simulink model "nelinerani_i_linearni_model_neupravljanog_objekta"  (R2018a)
settings: Solver=ode4  StartTime=0.0  StopTime=700  FixedStep=0.01  RelTol=1e-3  EnableMultiTasking=on
values from neighbouring files (symbols this model uses):
  Ar1 = 0.04    [skript_prvi_deo.m]
  Ar2 = 0.04    [skript_prvi_deo.m]
  Cd1 = 0.65    [skript_prvi_deo.m]
  Cd2 = 0.65    [skript_prvi_deo.m]
  Cdh = 0.65    [skript_prvi_deo.m]
  Cdt = 0.65    [skript_prvi_deo.m]
  df1_H1 = double(subs(df1_H1, [Uvt Uvh Uv2 Pt H1 H2 theta_m], [Uvt_N Uvh_N Uv2_N Pt_N H1_N H2_N theta_m_N]))    [skript_prvi_deo.m]
  df1_Pt = double(subs(df1_Pt, [Uvt Uvh Uv2 Pt H1 H2 theta_m], [Uvt_N Uvh_N Uv2_N Pt_N H1_N H2_N theta_m_N]))    [skript_prvi_deo.m]
  df1_Uvh = double(subs(df1_Uvh, [Uvt Uvh Uv2 Pt H1 H2 theta_m], [Uvt_N Uvh_N Uv2_N Pt_N H1_N H2_N theta_m_N]))    [skript_prvi_deo.m]
  df1_Uvt = double(subs(df1_Uvt, [Uvt Uvh Uv2 Pt H1 H2 theta_m], [Uvt_N Uvh_N Uv2_N Pt_N H1_N H2_N theta_m_N]))    [skript_prvi_deo.m]
  df2_H1 = double(subs(df2_H1, [Uvt Uvh Uv2 Pt H1 H2 theta_m], [Uvt_N Uvh_N Uv2_N Pt_N H1_N H2_N theta_m_N]))    [skript_prvi_deo.m]
  df2_H2 = double(subs(df2_H2, [Uvt Uvh Uv2 Pt H1 H2 theta_m], [Uvt_N Uvh_N Uv2_N Pt_N H1_N H2_N theta_m_N]))    [skript_prvi_deo.m]
  df2_Uv2 = double(subs(df2_Uv2, [Uvt Uvh Uv2 Pt H1 H2 theta_m], [Uvt_N Uvh_N Uv2_N Pt_N H1_N H2_N theta_m_N]))    [skript_prvi_deo.m]
  df3_H1 = double(subs(df3_H1, [Uvt Uvh Uv2 Pt H1 H2 theta_m], [Uvt_N Uvh_N Uv2_N Pt_N H1_N H2_N theta_m_N]))    [skript_prvi_deo.m]
  df3_Pt = double(subs(df3_Pt, [Uvt Uvh Uv2 Pt H1 H2 theta_m], [Uvt_N Uvh_N Uv2_N Pt_N H1_N H2_N theta_m_N]))    [skript_prvi_deo.m]
  df3_theta_m = double(subs(df3_theta_m, [Uvt Uvh Uv2 Pt H1 H2 theta_m], [Uvt_N Uvh_N Uv2_N Pt_N H1_N H2_N theta_m_N]))    [skript_prvi_deo.m]
  df3_Uvh = double(subs(df3_Uvh, [Uvt Uvh Uv2 Pt H1 H2 theta_m], [Uvt_N Uvh_N Uv2_N Pt_N H1_N H2_N theta_m_N]))    [skript_prvi_deo.m]
  df3_Uvt = double(subs(df3_Uvt, [Uvt Uvh Uv2 Pt H1 H2 theta_m], [Uvt_N Uvh_N Uv2_N Pt_N H1_N H2_N theta_m_N]))    [skript_prvi_deo.m]
  g = 9.81    [skript_prvi_deo.m]
  H1_max = 1.5    [skript_prvi_deo.m]
  H1_min = 0    [skript_prvi_deo.m]
  H1_N = 0.7    [skript_prvi_deo.m]
  H2_max = 1.5    [skript_prvi_deo.m]
  H2_min = 0    [skript_prvi_deo.m]
  H2_N = 0.8    [skript_prvi_deo.m]
  Kv1 = 1.5/1000    (= 0.0015)    [skript_prvi_deo.m]
  Kv2 = 1.5/1000    (= 0.0015)    [skript_prvi_deo.m]
  Kvh = 1/1000    (= 0.001)    [skript_prvi_deo.m]
  Kvt = 1/1000    (= 0.001)    [skript_prvi_deo.m]
  Ph = 3.25*10^5    (= 325000)    [skript_prvi_deo.m]
  Pt_N = 3.25*10^5    (= 325000)    [skript_prvi_deo.m]
  ro = 1000    [skript_prvi_deo.m]
  theta_h = 10 + 273    (= 283)    [skript_prvi_deo.m]
  theta_m_N = 30 + 273    (= 303)    [skript_prvi_deo.m]
  theta_t = 70 + 273    (= 343)    [skript_prvi_deo.m]
  Uv1 = 3    [skript_prvi_deo.m]
  Uv2_max = 10    [skript_prvi_deo.m]
  Uv2_min = 0    [skript_prvi_deo.m]
  Uv2_N = double(solve(e3 == 0, U2_N))    [skript_prvi_deo.m]
  Uvh_max = 10    [skript_prvi_deo.m]
  Uvh_min = 0    [skript_prvi_deo.m]
  Uvh_N = double(solve(f1n == 0, Uh_N))    [skript_prvi_deo.m]
  Uvt_max = 10    [skript_prvi_deo.m]
  Uvt_min = 0    [skript_prvi_deo.m]
  Uvt_N = double(solve(sol1 == sol2, Uvt_N))    [skript_prvi_deo.m]
  w1 = 0.1    [skript_prvi_deo.m]
  w2 = 0.1    [skript_prvi_deo.m]
  wh = 0.03    [skript_prvi_deo.m]
  wt = 0.03    [skript_prvi_deo.m]
settings Model: Creator=Nikola  LastModifiedBy=lakim
settings DataIOCC: LimitDataPoints=on  SaveFormat=Array
settings OptimizationCC: LifeSpan=inf
settings DebuggingCC: SFUnexpectedBacktrackingDiag=warning  SFNoUnconditionalDefaultTransitionDiag=warning  SFExecutionAtInitializationDiag=none
settings HardwareCC: ProdBitPerPointer=32  ProdBitPerSizeT=32  ProdBitPerPtrDiffT=32  ProdLargestAtomicFloat=None  ProdIntDivRoundTo=Undefined  ProdEndianess=Unspecified  ProdWordSize=32  ProdHWDeviceType=32-bit Generic
settings ModelReferenceCC: PropagateSignalLabelsOutOfModel=off
settings CodeAppCC: StateflowObjectComments=on
settings GRTTargetCC: TargetLangStandard=C89/C90 (ANSI)  GeneratePreprocessorConditionals=Disable all
settings ConfigComp: CovMetricSettings=dw  CovHtmlReporting=on  CovSaveCumulativeToWorkspaceVar=on  CovSaveSingleToWorkspaceVar=on  CovExternalEMLEnable=off

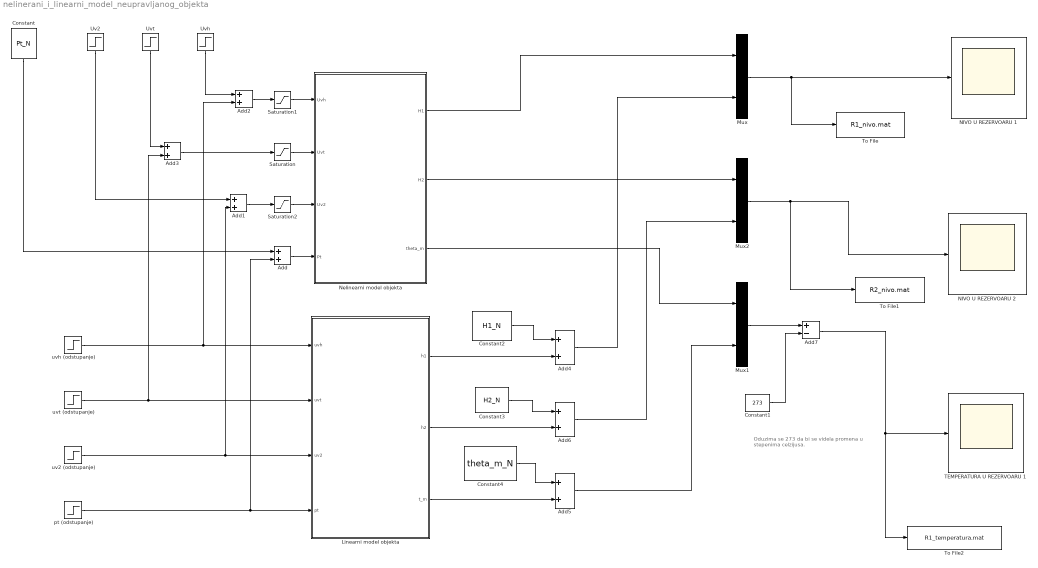
== system nelinerani_i_linearni_model_neupravljanog_objekta ==
  note: Oduzima se 273 da
      | bi se videla promena
      | u stepenima celzijusa.
  Add{,1..6} (7 alike) : Sum
  Add7 : Sum  Inputs=+-
  Constant : Constant  Value=Pt_N
  Constant1 : Constant  Value=273
  Constant2 : Constant  Value=H1_N
  Constant3 : Constant  Value=H2_N
  Constant4 : Constant  Value=theta_m_N
  Linearni model objekta : Subsystem
  Mux : Mux  Inputs=2
  Mux1 : Mux  Inputs=2
  Mux2 : Mux  Inputs=2
  NIVO U REZERVOARU 1 : Scope
  NIVO U REZERVOARU 2 : Scope
  Nelinearni model objekta : Subsystem
  Saturation : Saturate  UpperLimit=Uvt_max  LowerLimit=Uvt_min
  Saturation1 : Saturate  UpperLimit=Uvh_max  LowerLimit=Uvh_min
  Saturation2 : Saturate  UpperLimit=Uv2_max  LowerLimit=Uv2_min
  TEMPERATURA U REZERVOARU 1 : Scope
  To File : ToFile  Filename=R1_nivo.mat  MatrixName=H1
  To File1 : ToFile  Filename=R2_nivo.mat  MatrixName=H2
  To File2 : ToFile  Filename=R1_temperatura.mat  MatrixName=theta
  Uv2 : Step  Time=0  After=Uv2_N  SampleTime=0
  Uvh : Step  Time=0  After=Uvh_N  SampleTime=0
  Uvt : Step  Time=0  After=Uvt_N  SampleTime=0
  pt (odstupanje) : Step  Time=0  After=10^3  SampleTime=0
  uv2 (odstupanje) : Step  Time=0  After=0  SampleTime=0
  uvh (odstupanje) : Step  Time=150  After=0.1  SampleTime=0
  uvt (odstupanje) : Step  Time=0  After=0  SampleTime=0
  wires:
  Constant/1 -> Add/1
  Add3/1 -> Saturation/1
  Uvt/1 -> Add3/1
  Uvh/1 -> Add2/1
  Uv2/1 -> Add1/1
  Nelinearni model objekta/1(H1) -> Mux/1
  Mux/1 -> To File/1, NIVO U REZERVOARU 1/1
  Nelinearni model objekta/2(H2) -> Mux2/1
  Mux2/1 -> To File1/1, NIVO U REZERVOARU 2/1
  Nelinearni model objekta/3(theta_m) -> Mux1/1
  Add2/1 -> Saturation1/1
  Saturation/1 -> Nelinearni model objekta/2(Uvt)
  Add1/1 -> Saturation2/1
  uvh (odstupanje)/1 -> Add2/2, Linearni model objekta/1(uvh)
  uvt (odstupanje)/1 -> Add3/2, Linearni model objekta/2(uvt)
  uv2 (odstupanje)/1 -> Linearni model objekta/3(uv2), Add1/2
  pt (odstupanje)/1 -> Linearni model objekta/4(pt), Add/2
  Linearni model objekta/1(h1) -> Add4/2
  Linearni model objekta/2(h2) -> Add6/2
  Linearni model objekta/3(t_m) -> Add5/2
  Constant4/1 -> Add5/1
  Constant3/1 -> Add6/1
  Constant2/1 -> Add4/1
  Add4/1 -> Mux/2
  Add6/1 -> Mux2/2
  Add5/1 -> Mux1/2
  Add/1 -> Nelinearni model objekta/4(Pt)
  Saturation1/1 -> Nelinearni model objekta/1(Uvh)
  Saturation2/1 -> Nelinearni model objekta/3(Uv2)
  Mux1/1 -> Add7/1
  Add7/1 -> To File2/1, TEMPERATURA U REZERVOARU 1/1
  Constant1/1 -> Add7/2

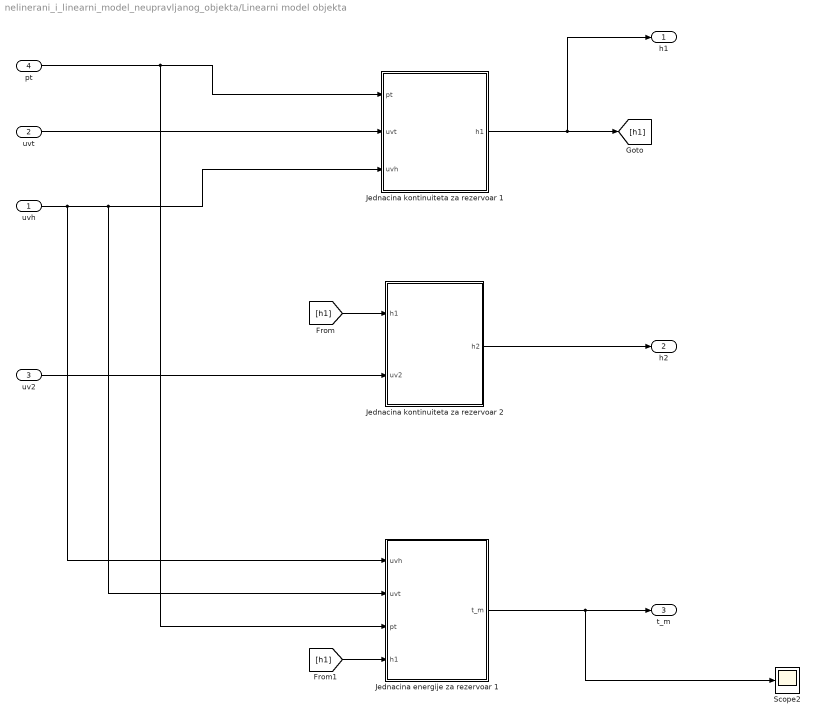
== system nelinerani_i_linearni_model_neupravljanog_objekta/Linearni model objekta ==
  uvh : Inport
  uvt : Inport  Port=2
  uv2 : Inport  Port=3
  pt : Inport  Port=4
  Jednacina energije za rezervoar 1 : Subsystem
  Jednacina kontinuiteta za rezervoar 1 : Subsystem
  Jednacina kontinuiteta za rezervoar 2 : Subsystem
  Scope2 : Scope
  h1 : Outport
  h2 : Outport  Port=2
  t_m : Outport  Port=3
  wires:
  Jednacina kontinuiteta za rezervoar 1/1(h1) -> h1/1, [h1]
  [h1] -> Jednacina kontinuiteta za rezervoar 2/1(h1)
  Jednacina kontinuiteta za rezervoar 2/1(h2) -> h2/1
  Jednacina energije za rezervoar 1/1(t_m) -> Scope2/1, t_m/1
  pt/1 -> Jednacina energije za rezervoar 1/3(pt), Jednacina kontinuiteta za rezervoar 1/1(pt)
  uvt/1 -> Jednacina kontinuiteta za rezervoar 1/2(uvt)
  uvh/1 -> Jednacina energije za rezervoar 1/1(uvh), Jednacina energije za rezervoar 1/2(uvt), Jednacina kontinuiteta za rezervoar 1/3(uvh)
  uv2/1 -> Jednacina kontinuiteta za rezervoar 2/2(uv2)
  [h1] -> Jednacina energije za rezervoar 1/4(h1)

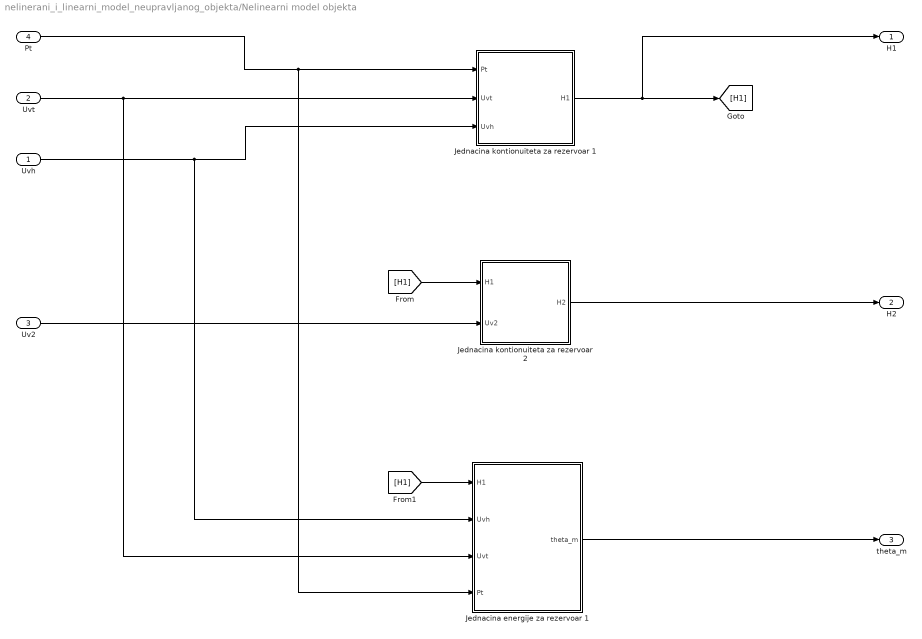
== system nelinerani_i_linearni_model_neupravljanog_objekta/Nelinearni model objekta ==
  Uvh : Inport
  Uvt : Inport  Port=2
  Uv2 : Inport  Port=3
  Pt : Inport  Port=4
  Jednacina energije za rezervoar 1 : Subsystem
  Jednacina kontionuiteta za rezervoar 1 : Subsystem
  Jednacina kontionuiteta za rezervoar 2 : Subsystem
  H1 : Outport
  H2 : Outport  Port=2
  theta_m : Outport  Port=3
  wires:
  Jednacina kontionuiteta za rezervoar 1/1(H1) -> [H1], H1/1
  [H1] -> Jednacina energije za rezervoar 1/1(H1)
  Uvh/1 -> Jednacina energije za rezervoar 1/2(Uvh), Jednacina kontionuiteta za rezervoar 1/3(Uvh)
  Uvt/1 -> Jednacina energije za rezervoar 1/3(Uvt), Jednacina kontionuiteta za rezervoar 1/2(Uvt)
  Pt/1 -> Jednacina energije za rezervoar 1/4(Pt), Jednacina kontionuiteta za rezervoar 1/1(Pt)
  Uv2/1 -> Jednacina kontionuiteta za rezervoar 2/2(Uv2)
  Jednacina kontionuiteta za rezervoar 2/1(H2) -> H2/1
  Jednacina energije za rezervoar 1/1(theta_m) -> theta_m/1
  [H1] -> Jednacina kontionuiteta za rezervoar 2/1(H1)

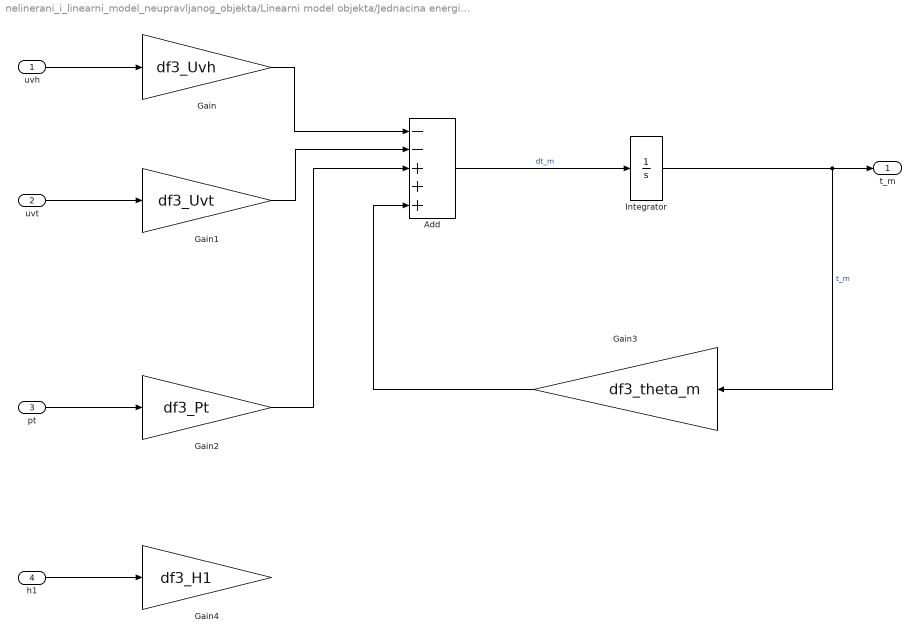
== system nelinerani_i_linearni_model_neupravljanog_objekta/Linearni model objekta/Jednacina energije za rezervoar 1 ==
  uvh : Inport
  uvt : Inport  Port=2
  pt : Inport  Port=3
  h1 : Inport  Port=4
  Add : Sum  Inputs=--+++
  Gain : Gain  Gain=df3_Uvh
  Gain1 : Gain  Gain=df3_Uvt
  Gain2 : Gain  Gain=df3_Pt
  Gain3 : Gain  Gain=df3_theta_m
  Gain4 : Gain  Gain=df3_H1
  Integrator : Integrator
  t_m : Outport
  wires:
  Add/1 -> Integrator/1  "dt_m"
  Integrator/1 -> Gain3/1, t_m/1  "t_m"
  uvh/1 -> Gain/1
  Gain/1 -> Add/1
  uvt/1 -> Gain1/1
  Gain1/1 -> Add/2
  pt/1 -> Gain2/1
  Gain2/1 -> Add/3
  h1/1 -> Gain4/1
  Gain3/1 -> Add/5

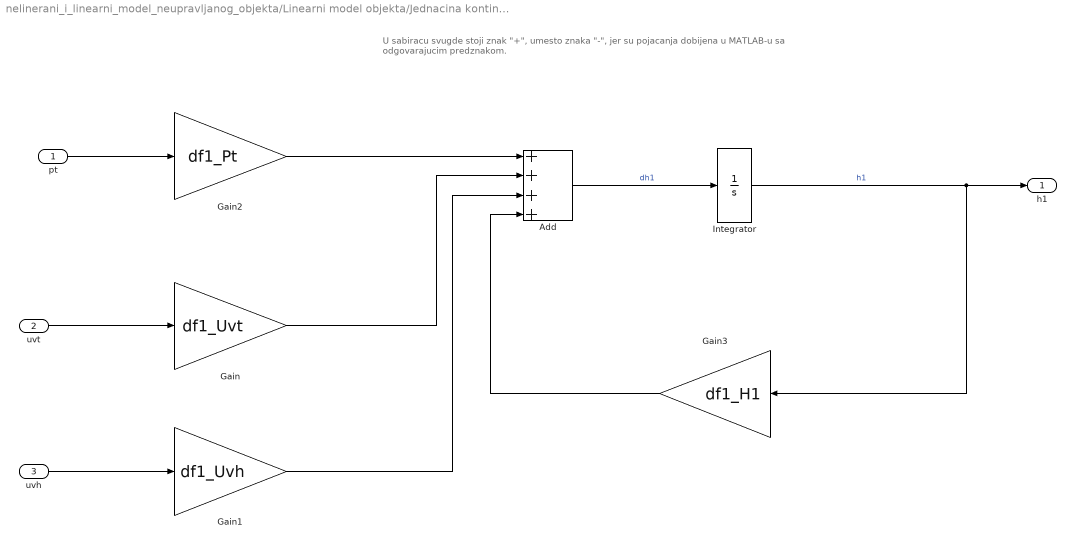
== system nelinerani_i_linearni_model_neupravljanog_objekta/Linearni model objekta/Jednacina kontinuiteta za rezervoar 1 ==
  note: U sabiracu svugde stoji znak "+", umesto znaka "-", jer
      | su pojacanja dobijena u MATLAB-u sa
      | odgovarajucim predznakom.
  pt : Inport
  uvt : Inport  Port=2
  uvh : Inport  Port=3
  Add : Sum  Inputs=++++
  Gain : Gain  Gain=df1_Uvt
  Gain1 : Gain  Gain=df1_Uvh
  Gain2 : Gain  Gain=df1_Pt
  Gain3 : Gain  Gain=df1_H1
  Integrator : Integrator
  h1 : Outport
  wires:
  pt/1 -> Gain2/1
  uvt/1 -> Gain/1
  uvh/1 -> Gain1/1
  Add/1 -> Integrator/1  "dh1"
  Integrator/1 -> Gain3/1, h1/1  "h1"
  Gain2/1 -> Add/1
  Gain/1 -> Add/2
  Gain1/1 -> Add/3
  Gain3/1 -> Add/4

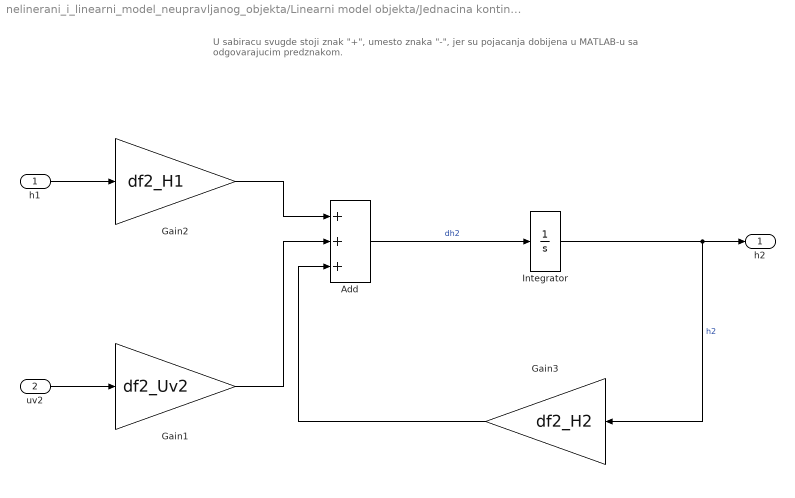
== system nelinerani_i_linearni_model_neupravljanog_objekta/Linearni model objekta/Jednacina kontinuiteta za rezervoar 2 ==
  note: U sabiracu svugde stoji znak "+", umesto znaka "-", jer
      | su pojacanja dobijena u MATLAB-u sa
      | odgovarajucim predznakom.
  h1 : Inport
  uv2 : Inport  Port=2
  Add : Sum  Inputs=+++
  Gain1 : Gain  Gain=df2_Uv2
  Gain2 : Gain  Gain=df2_H1
  Gain3 : Gain  Gain=df2_H2
  Integrator : Integrator
  h2 : Outport
  wires:
  Add/1 -> Integrator/1  "dh2"
  h1/1 -> Gain2/1
  Gain2/1 -> Add/1
  uv2/1 -> Gain1/1
  Gain1/1 -> Add/2
  Integrator/1 -> Gain3/1, h2/1  "h2"
  Gain3/1 -> Add/3

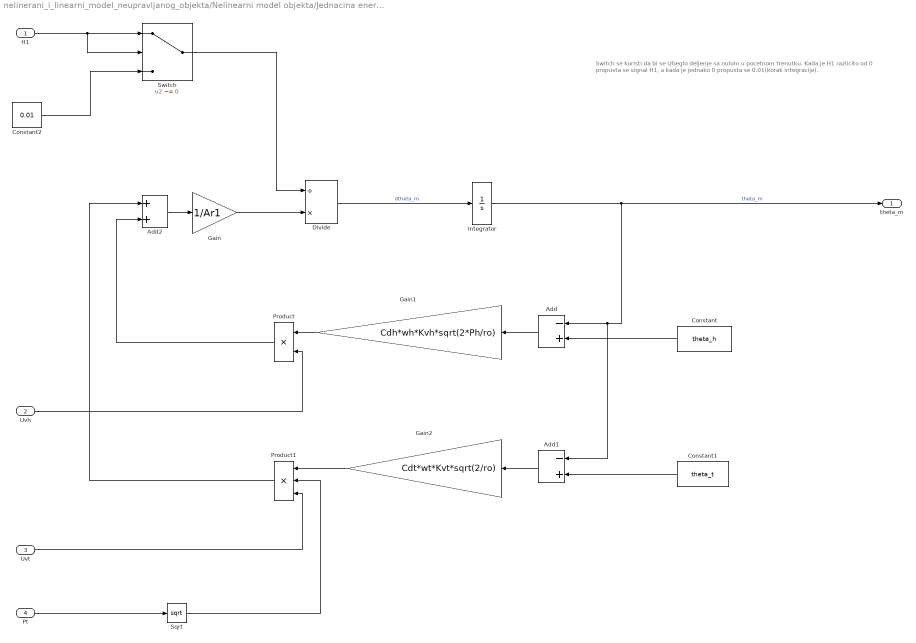
== system nelinerani_i_linearni_model_neupravljanog_objekta/Nelinearni model objekta/Jednacina energije za rezervoar 1 ==
  note: Switch se koristi da bi se izbeglo deljenje sa nulom
      | u pocetnom trenutku. Kada je H1 razlicito od 0 propusta se
      | signal H1, a kada je jednako 0 propusta se 0.01(korak integracije).
  H1 : Inport
  Uvh : Inport  Port=2
  Uvt : Inport  Port=3
  Pt : Inport  Port=4
  Add : Sum  Inputs=-+
  Add1 : Sum  Inputs=-+
  Add2 : Sum
  Constant : Constant  Value=theta_h
  Constant1 : Constant  Value=theta_t
  Constant2 : Constant  Value=0.01
  Divide : Product  Inputs=/*
  Gain : Gain  Gain=1/Ar1
  Gain1 : Gain  Gain=Cdh*wh*Kvh*sqrt(2*Ph/ro)
  Gain2 : Gain  Gain=Cdt*wt*Kvt*sqrt(2/ro)
  Integrator : Integrator  InitialCondition=theta_m_N
  Product : Product
  Product1 : Product  Inputs=3
  Sqrt : Sqrt  SaturateOnIntegerOverflow=on
  Switch : Switch  Criteria=u2 ~= 0
  theta_m : Outport
  wires:
  Integrator/1 -> Add1/1, Add/1, theta_m/1  "theta_m"
  Constant/1 -> Add/2
  Constant1/1 -> Add1/2
  Add/1 -> Gain1/1
  Gain1/1 -> Product/1
  Uvh/1 -> Product/2
  Add1/1 -> Gain2/1
  Gain2/1 -> Product1/1
  Pt/1 -> Sqrt/1
  Uvt/1 -> Product1/3
  Sqrt/1 -> Product1/2
  Product/1 -> Add2/2
  Product1/1 -> Add2/1
  Add2/1 -> Gain/1
  Divide/1 -> Integrator/1  "dtheta_m"
  H1/1 -> Switch/2, Switch/1
  Constant2/1 -> Switch/3
  Switch/1 -> Divide/1
  Gain/1 -> Divide/2

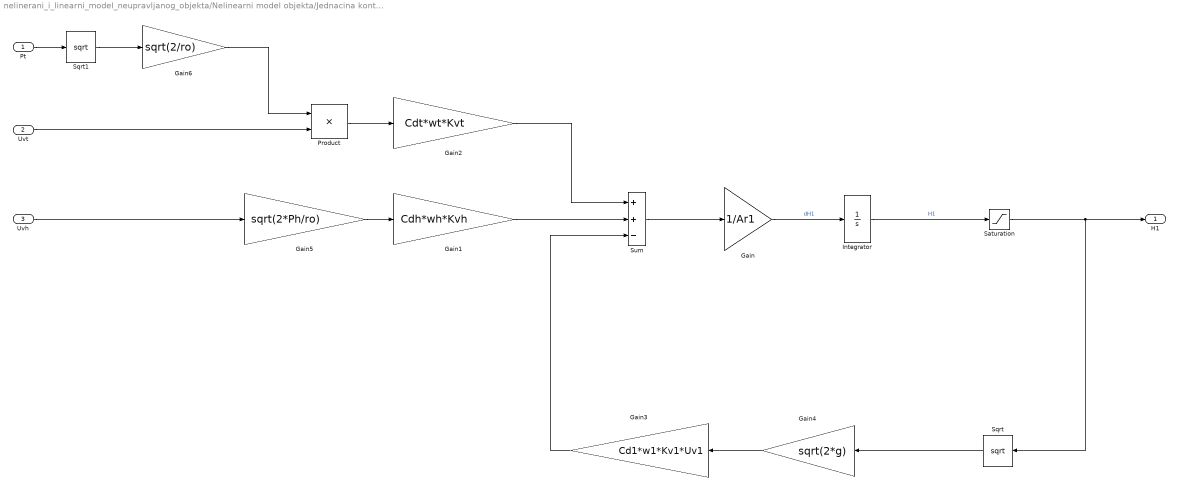
== system nelinerani_i_linearni_model_neupravljanog_objekta/Nelinearni model objekta/Jednacina kontionuiteta za rezervoar 1 ==
  Pt : Inport
  Uvt : Inport  Port=2
  Uvh : Inport  Port=3
  Gain : Gain  Gain=1/Ar1
  Gain1 : Gain  Gain=Cdh*wh*Kvh
  Gain2 : Gain  Gain=Cdt*wt*Kvt
  Gain3 : Gain  Gain=Cd1*w1*Kv1*Uv1
  Gain4 : Gain  Gain=sqrt(2*g)
  Gain5 : Gain  Gain=sqrt(2*Ph/ro)
  Gain6 : Gain  Gain=sqrt(2/ro)
  Integrator : Integrator  InitialCondition=H1_N
  Product : Product
  Saturation : Saturate  UpperLimit=H1_max  LowerLimit=H1_min
  Sqrt : Sqrt  SaturateOnIntegerOverflow=on
  Sqrt1 : Sqrt  SaturateOnIntegerOverflow=on
  Sum : Sum  Inputs=++-
  H1 : Outport
  wires:
  Gain/1 -> Integrator/1  "dH1"
  Sum/1 -> Gain/1
  Integrator/1 -> Saturation/1  "H1"
  Sqrt/1 -> Gain4/1
  Gain4/1 -> Gain3/1
  Gain3/1 -> Sum/3
  Gain1/1 -> Sum/2
  Gain2/1 -> Sum/1
  Gain5/1 -> Gain1/1
  Uvh/1 -> Gain5/1
  Pt/1 -> Sqrt1/1
  Uvt/1 -> Product/2
  Product/1 -> Gain2/1
  Sqrt1/1 -> Gain6/1
  Gain6/1 -> Product/1
  Saturation/1 -> Sqrt/1, H1/1

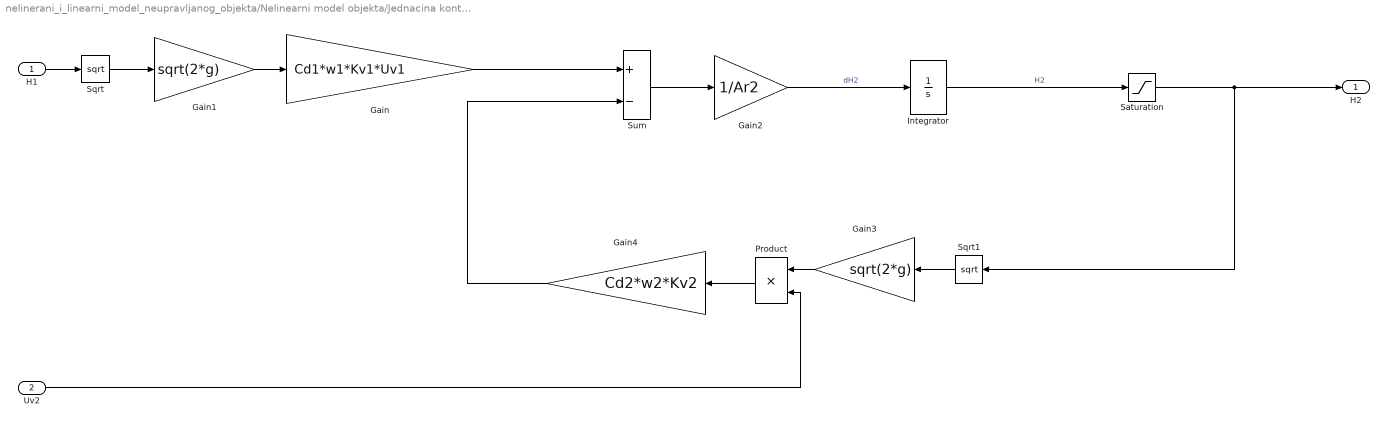
== system nelinerani_i_linearni_model_neupravljanog_objekta/Nelinearni model objekta/Jednacina kontionuiteta za rezervoar 2 ==
  H1 : Inport
  Uv2 : Inport  Port=2
  Gain : Gain  Gain=Cd1*w1*Kv1*Uv1
  Gain1 : Gain  Gain=sqrt(2*g)
  Gain2 : Gain  Gain=1/Ar2
  Gain3 : Gain  Gain=sqrt(2*g)
  Gain4 : Gain  Gain=Cd2*w2*Kv2
  Integrator : Integrator  InitialCondition=H2_N
  Product : Product
  Saturation : Saturate  UpperLimit=H2_max  LowerLimit=H2_min
  Sqrt : Sqrt  SaturateOnIntegerOverflow=on
  Sqrt1 : Sqrt  SaturateOnIntegerOverflow=on
  Sum : Sum  Inputs=+-
  H2 : Outport
  wires:
  H1/1 -> Sqrt/1
  Sqrt/1 -> Gain1/1
  Gain1/1 -> Gain/1
  Gain/1 -> Sum/1
  Sum/1 -> Gain2/1
  Gain2/1 -> Integrator/1  "dH2"
  Integrator/1 -> Saturation/1  "H2"
  Sqrt1/1 -> Gain3/1
  Gain3/1 -> Product/1
  Uv2/1 -> Product/2
  Product/1 -> Gain4/1
  Gain4/1 -> Sum/2
  Saturation/1 -> Sqrt1/1, H2/1
